simulink model "MGmono_rtiFPGASeparationFile"  (R2018b)
settings: Solver=FixedStepAuto  StartTime=0.0  StopTime=Inf  FixedStep=N*T  RelTol=1e-3
PostLoadFcn:
  | , if any(exist('dsrtsu_mdlpostloadfcn', 'file') ~= 0), dsrtsu_mdlpostloadfcn('Execute', bdroot); end,
InitFcn:
  | , if any(exist('dsmpb_private', 'file') ~= 0), dsmpb_private('dsmpb_mdlclblib', 'Init', bdroot); end,
values from neighbouring files (symbols this model uses):
  amp = 1    [param.m]
  fixedgain_i = 10*1000/(3*100)    (= 33.3333333333)    [param.m]
  fixedgain_vc1 = 10*10000/(3*100*2.5)    (= 133.333333333)    [param.m]
  fixedgain_vc2 = 10*10000/(3*100*2.5)    (= 133.333333333)    [param.m]
  fixedgain_vc3 = 10*22000/(3*100*2.5)    (= 293.333333333)    [param.m]
  fixedgain_vc4 = 10*22000/(3*100*2.5)    (= 293.333333333)    [param.m]
  fixedgain_vc5 = 10*22000/(3*100*2.5)    (= 293.333333333)    [param.m]
  freq = 50    [param.m]
  gain_iL1 = 1    [param.m]
  gain_iL2 = 1    [param.m]
  gain_iL3 = 1    [param.m]
  gain_iL4 = 1    [param.m]
  gain_vc1 = 1    [param.m]
  gain_vc2 = 1    [param.m]
  gain_vc3 = 1    [param.m]
  gain_vc4 = 1    [param.m]
  gain_vc5 = 1    [param.m]
  Ii = 10    [param.m]
  Ipv = 0.01    [param.m]
  Iv = 0.1    [param.m]
  Ki = 1e-7    (= 1e-07)    [param.m]
  Kp = 0.5    [param.m]
  maxd = N-1    (= 9)    [param.m]
  mind = 1    [param.m]
  N = 10    [param.m]
  offset_iL1 = 0.2    [param.m]
  offset_iL2 = 0.2    [param.m]
  offset_iL3 = -2e-3    (= -0.002)    [param.m]
  offset_iL4 = -2e-3    (= -0.002)    [param.m]
  offset_vc1 = -0.21    [param.m]
  offset_vc2 = -0.17    [param.m]
  offset_vc3 = 0.2    [param.m]
  offset_vc4 = -0.05    [param.m]
  offset_vc5 = -0.01    [param.m]
  Pi = 0.3    [param.m]
  Ppv = 0.05    [param.m]
  Pv = 0.01    [param.m]
  T = 6e-6    (= 6e-06)    [param.m]
  Tf = 1/1000    (= 0.001)    [param.m]
  Tfdc = 1/20    (= 0.05)    [param.m]
  v_dc_ref = 80    [param.m]
undefined symbols (not defined in the file or in its folder): DiscIntNeverNeededParam
libraries: xbsIndex_r4 x155, rti1202lib_adc_class1 x9, rtiproclib x7, simulink x6, rtifpgainterfacelib x1
(part 5 of 5)

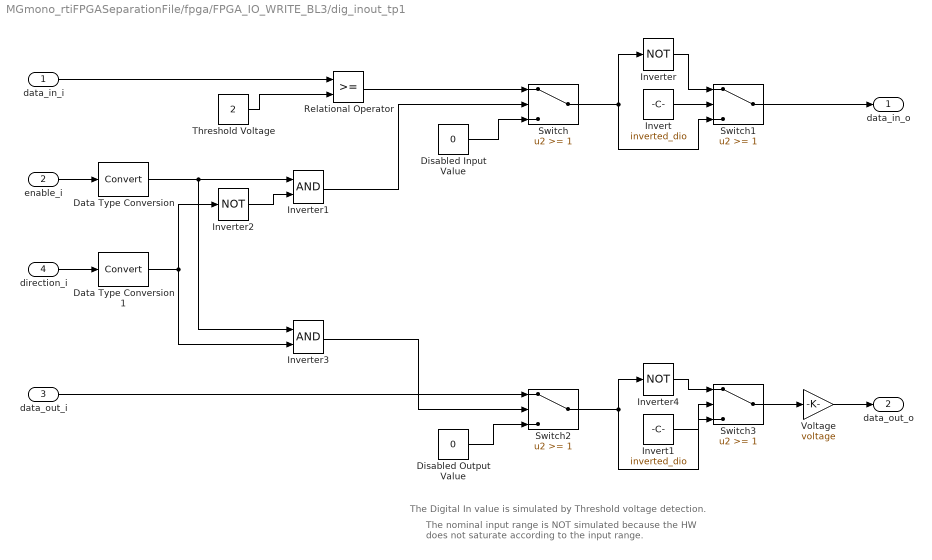
== system MGmono_rtiFPGASeparationFile/fpga/FPGA_IO_WRITE_BL3/dig_inout_tp1 ==
  note: The nominal input range is NOT simulated because
      | the HW does not saturate according to the input range.
  note: The Digital In value is simulated by Threshold voltage detection.
  data_in_i : Inport
  enable_i : Inport  Port=2
  data_out_i : Inport  Port=3
  direction_i : Inport  Port=4
  Data Type Conversion : DataTypeConversion
  Data Type Conversion1 : DataTypeConversion
  Disabled Input Value : Constant  Value=0
  Disabled Output Value : Constant  Value=0
  Invert : Constant  Value=inverted_dio
  Invert1 : Constant  Value=inverted_dio
  Inverter : Logic  Operator=NOT  AllPortsSameDT=off  OutDataTypeStr=boolean
  Inverter1 : Logic  AllPortsSameDT=off  OutDataTypeStr=boolean
  Inverter2 : Logic  Operator=NOT  AllPortsSameDT=off  OutDataTypeStr=boolean
  Inverter3 : Logic  AllPortsSameDT=off  OutDataTypeStr=boolean
  Inverter4 : Logic  Operator=NOT  AllPortsSameDT=off  OutDataTypeStr=boolean
  Relational Operator : RelationalOperator  OutDataTypeStr=boolean  RndMeth=Nearest
  Switch{,1..3} (4 alike) : Switch  Threshold=1
  Threshold Voltage : Constant  Value=2
  Voltage : Gain  Gain=voltage  ParamDataTypeStr=float('double')
  data_in_o : Outport
  data_out_o : Outport  Port=2
  wires:
  Voltage/1 -> data_out_o/1
  Data Type Conversion1/1 -> Inverter3/2, Inverter2/1
  Data Type Conversion/1 -> Inverter3/1, Inverter1/1
  Switch3/1 -> Voltage/1
  Switch2/1 -> Switch3/3, Inverter4/1
  Inverter4/1 -> Switch3/1
  Invert1/1 -> Switch3/2
  data_out_i/1 -> Switch2/1
  Inverter3/1 -> Switch2/2
  Disabled Output Value/1 -> Switch2/3
  Inverter2/1 -> Inverter1/2
  direction_i/1 -> Data Type Conversion1/1
  Inverter1/1 -> Switch/2
  enable_i/1 -> Data Type Conversion/1
  Switch/1 -> Switch1/3, Inverter/1
  Relational Operator/1 -> Switch/1
  Inverter/1 -> Switch1/1
  Invert/1 -> Switch1/2
  Switch1/1 -> data_in_o/1
  Disabled Input Value/1 -> Switch/3
  Threshold Voltage/1 -> Relational Operator/2
  data_in_i/1 -> Relational Operator/1

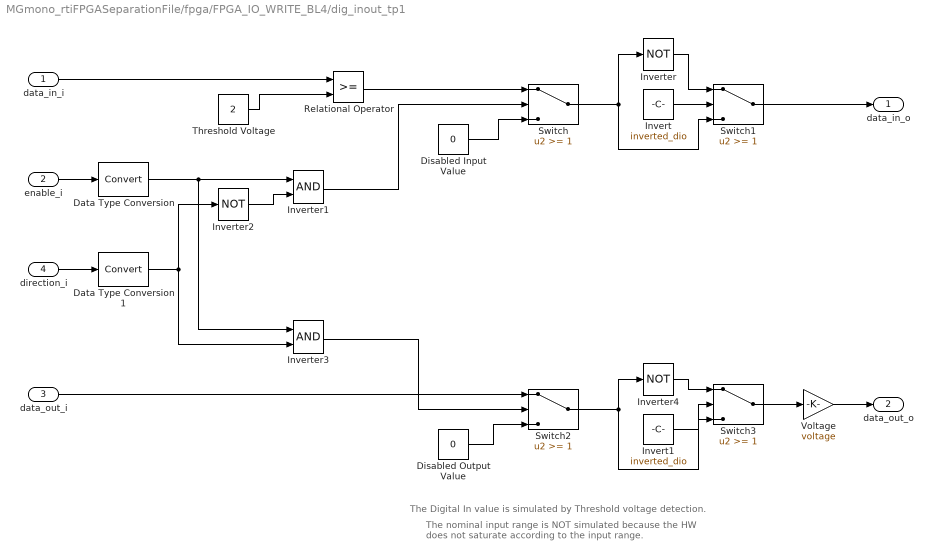
== system MGmono_rtiFPGASeparationFile/fpga/FPGA_IO_WRITE_BL4/dig_inout_tp1 ==
  note: The nominal input range is NOT simulated because
      | the HW does not saturate according to the input range.
  note: The Digital In value is simulated by Threshold voltage detection.
  data_in_i : Inport
  enable_i : Inport  Port=2
  data_out_i : Inport  Port=3
  direction_i : Inport  Port=4
  Data Type Conversion : DataTypeConversion
  Data Type Conversion1 : DataTypeConversion
  Disabled Input Value : Constant  Value=0
  Disabled Output Value : Constant  Value=0
  Invert : Constant  Value=inverted_dio
  Invert1 : Constant  Value=inverted_dio
  Inverter : Logic  Operator=NOT  AllPortsSameDT=off  OutDataTypeStr=boolean
  Inverter1 : Logic  AllPortsSameDT=off  OutDataTypeStr=boolean
  Inverter2 : Logic  Operator=NOT  AllPortsSameDT=off  OutDataTypeStr=boolean
  Inverter3 : Logic  AllPortsSameDT=off  OutDataTypeStr=boolean
  Inverter4 : Logic  Operator=NOT  AllPortsSameDT=off  OutDataTypeStr=boolean
  Relational Operator : RelationalOperator  OutDataTypeStr=boolean  RndMeth=Nearest
  Switch{,1..3} (4 alike) : Switch  Threshold=1
  Threshold Voltage : Constant  Value=2
  Voltage : Gain  Gain=voltage  ParamDataTypeStr=float('double')
  data_in_o : Outport
  data_out_o : Outport  Port=2
  wires:
  Voltage/1 -> data_out_o/1
  Data Type Conversion1/1 -> Inverter3/2, Inverter2/1
  Data Type Conversion/1 -> Inverter3/1, Inverter1/1
  Switch3/1 -> Voltage/1
  Switch2/1 -> Switch3/3, Inverter4/1
  Inverter4/1 -> Switch3/1
  Invert1/1 -> Switch3/2
  data_out_i/1 -> Switch2/1
  Inverter3/1 -> Switch2/2
  Disabled Output Value/1 -> Switch2/3
  Inverter2/1 -> Inverter1/2
  direction_i/1 -> Data Type Conversion1/1
  Inverter1/1 -> Switch/2
  enable_i/1 -> Data Type Conversion/1
  Switch/1 -> Switch1/3, Inverter/1
  Relational Operator/1 -> Switch/1
  Inverter/1 -> Switch1/1
  Invert/1 -> Switch1/2
  Switch1/1 -> data_in_o/1
  Disabled Input Value/1 -> Switch/3
  Threshold Voltage/1 -> Relational Operator/2
  data_in_i/1 -> Relational Operator/1

== system MGmono_rtiFPGASeparationFile/fpga/FPGA_IO_WRITE_BL5/dig_inout_tp1 ==
  note: The nominal input range is NOT simulated because
      | the HW does not saturate according to the input range.
  note: The Digital In value is simulated by Threshold voltage detection.
  data_in_i : Inport
  enable_i : Inport  Port=2
  data_out_i : Inport  Port=3
  direction_i : Inport  Port=4
  Data Type Conversion : DataTypeConversion
  Data Type Conversion1 : DataTypeConversion
  Disabled Input Value : Constant  Value=0
  Disabled Output Value : Constant  Value=0
  Invert : Constant  Value=inverted_dio
  Invert1 : Constant  Value=inverted_dio
  Inverter : Logic  Operator=NOT  AllPortsSameDT=off  OutDataTypeStr=boolean
  Inverter1 : Logic  AllPortsSameDT=off  OutDataTypeStr=boolean
  Inverter2 : Logic  Operator=NOT  AllPortsSameDT=off  OutDataTypeStr=boolean
  Inverter3 : Logic  AllPortsSameDT=off  OutDataTypeStr=boolean
  Inverter4 : Logic  Operator=NOT  AllPortsSameDT=off  OutDataTypeStr=boolean
  Relational Operator : RelationalOperator  OutDataTypeStr=boolean  RndMeth=Nearest
  Switch{,1..3} (4 alike) : Switch  Threshold=1
  Threshold Voltage : Constant  Value=2
  Voltage : Gain  Gain=voltage  ParamDataTypeStr=float('double')
  data_in_o : Outport
  data_out_o : Outport  Port=2
  wires:
  Voltage/1 -> data_out_o/1
  Data Type Conversion1/1 -> Inverter3/2, Inverter2/1
  Data Type Conversion/1 -> Inverter3/1, Inverter1/1
  Switch3/1 -> Voltage/1
  Switch2/1 -> Switch3/3, Inverter4/1
  Inverter4/1 -> Switch3/1
  Invert1/1 -> Switch3/2
  data_out_i/1 -> Switch2/1
  Inverter3/1 -> Switch2/2
  Disabled Output Value/1 -> Switch2/3
  Inverter2/1 -> Inverter1/2
  direction_i/1 -> Data Type Conversion1/1
  Inverter1/1 -> Switch/2
  enable_i/1 -> Data Type Conversion/1
  Switch/1 -> Switch1/3, Inverter/1
  Relational Operator/1 -> Switch/1
  Inverter/1 -> Switch1/1
  Invert/1 -> Switch1/2
  Switch1/1 -> data_in_o/1
  Disabled Input Value/1 -> Switch/3
  Threshold Voltage/1 -> Relational Operator/2
  data_in_i/1 -> Relational Operator/1

== system MGmono_rtiFPGASeparationFile/fpga/FPGA_XDATA_READ_BL1/phs_read_register ==
  note: Subsystem simulating the phs bus
      | access via RTLib functions.
  note: Subsystem simulating the communication
      | function specific behaviour. This is how the
      | FPGA framework driver takes effect on the data.
  data_i : Inport
  com_fct_model : Subsystem
  phs/rtlib_sim_model : Subsystem
  data_o : Outport
  data_new_o : Outport  Port=2
  wires:
  com_fct_model/2(data_new_o) -> data_new_o/1
  phs/rtlib_sim_model/1(data_o1) -> com_fct_model/1(data_i1)
  com_fct_model/1(data_o1) -> data_o/1
  data_i/1 -> phs/rtlib_sim_model/1(data_i1)

== system MGmono_rtiFPGASeparationFile/fpga/FPGA_XDATA_READ_BL2/phs_read_register ==
  note: Subsystem simulating the phs bus
      | access via RTLib functions.
  note: Subsystem simulating the communication
      | function specific behaviour. This is how the
      | FPGA framework driver takes effect on the data.
  data_i : Inport
  com_fct_model : Subsystem
  phs/rtlib_sim_model : Subsystem
  data_o : Outport
  data_new_o : Outport  Port=2
  wires:
  com_fct_model/2(data_new_o) -> data_new_o/1
  phs/rtlib_sim_model/1(data_o1) -> com_fct_model/1(data_i1)
  com_fct_model/1(data_o1) -> data_o/1
  data_i/1 -> phs/rtlib_sim_model/1(data_i1)

== system MGmono_rtiFPGASeparationFile/fpga/FPGA_XDATA_READ_BL3/phs_read_register ==
  note: Subsystem simulating the phs bus
      | access via RTLib functions.
  note: Subsystem simulating the communication
      | function specific behaviour. This is how the
      | FPGA framework driver takes effect on the data.
  data_i : Inport
  com_fct_model : Subsystem
  phs/rtlib_sim_model : Subsystem
  data_o : Outport
  data_new_o : Outport  Port=2
  wires:
  com_fct_model/2(data_new_o) -> data_new_o/1
  phs/rtlib_sim_model/1(data_o1) -> com_fct_model/1(data_i1)
  com_fct_model/1(data_o1) -> data_o/1
  data_i/1 -> phs/rtlib_sim_model/1(data_i1)

== system MGmono_rtiFPGASeparationFile/RTI Data/RTI Data Store/RTI Data Store/RTI Data Store ==
  RTI Data Store : Subsystem  mask(RTI_DATA_STORE){}
      mask help:
      | RTI Data Store Block. This block is used by RTI to store internal model dependent data. Deleting this block will result in data loss.
      |
      | NEVER DELETE, COPY, OR MODIFY THIS BLOCK!
      mask Help:
      | RTI Data Store Block. This block is used by RTI to store internal model dependent data. Deleting this block will result in data loss.
      | 
      | NEVER DELETE, COPY, OR MODIFY THIS BLOCK!
      mask Display: text(0.5, 0.5, ' ', 'HorizontalAlignment', 'center');

== system MGmono_rtiFPGASeparationFile/fpga/FPGA_INT_BL1/phs_interrupt/com_fct_model ==
  data_i1 : Inport
  data_o1 : Outport
  wires:
  data_i1/1 -> data_o1/1

== system MGmono_rtiFPGASeparationFile/fpga/FPGA_INT_BL1/phs_interrupt/phs//rtlib_sim_model ==
  note: - Detect the interrupt (rising edge).
      | - Generate function call.
  data_i1 : Inport
  Triggered Subsystem : Subsystem  TreatAsAtomicUnit=on
  data_o1 : Outport
  wires:
  Triggered Subsystem/1(Out1) -> data_o1/1
  data_i1/1 -> Triggered Subsystem/Trigger

== system MGmono_rtiFPGASeparationFile/fpga/FPGA_INT_BL2/phs_interrupt/com_fct_model ==
  data_i1 : Inport
  data_o1 : Outport
  wires:
  data_i1/1 -> data_o1/1

== system MGmono_rtiFPGASeparationFile/fpga/FPGA_INT_BL2/phs_interrupt/phs//rtlib_sim_model ==
  note: - Detect the interrupt (rising edge).
      | - Generate function call.
  data_i1 : Inport
  Triggered Subsystem : Subsystem  TreatAsAtomicUnit=on
  data_o1 : Outport
  wires:
  Triggered Subsystem/1(Out1) -> data_o1/1
  data_i1/1 -> Triggered Subsystem/Trigger

== system MGmono_rtiFPGASeparationFile/fpga/FPGA_INT_BL3/phs_interrupt/com_fct_model ==
  data_i1 : Inport
  data_o1 : Outport
  wires:
  data_i1/1 -> data_o1/1

== system MGmono_rtiFPGASeparationFile/fpga/FPGA_INT_BL3/phs_interrupt/phs//rtlib_sim_model ==
  note: - Detect the interrupt (rising edge).
      | - Generate function call.
  data_i1 : Inport
  Triggered Subsystem : Subsystem  TreatAsAtomicUnit=on
  data_o1 : Outport
  wires:
  Triggered Subsystem/1(Out1) -> data_o1/1
  data_i1/1 -> Triggered Subsystem/Trigger

== system MGmono_rtiFPGASeparationFile/fpga/FPGA_XDATA_READ_BL1/phs_read_register/com_fct_model ==
  note: - Register data is presented to the FPGA application without data adaptions.
      |
      | - Register group accesses are implicitly simulated by simulink: all FPGA
      | communication function interface blocks are simulated within one task
      | with a unique sample time --> in- and ouputs are sampled simultaneously
      | and therefore data consistency is guaranteed.
  data_i1 : Inport
  Data_New_Calc : Subsystem
  Zero-Order Hold : ZeroOrderHold  SampleTime=fpga_sample_time
  data_o1 : Outport
  data_new_o : Outport  Port=2
  wires:
  Zero-Order Hold/1 -> data_o1/1
  Data_New_Calc/1(Out1) -> data_new_o/1
  data_i1/1 -> Zero-Order Hold/1, Data_New_Calc/1(In1)

== system MGmono_rtiFPGASeparationFile/fpga/FPGA_XDATA_READ_BL1/phs_read_register/phs//rtlib_sim_model ==
  note: - The double to fixed-point conversion done by the XSG gateway behaves differently
      | than the conversion done by the RTLib C-code. Therefore the C-Code behaviour
      | is simulated via an s-function using the RTLib conversion technique including scaling and saturation.
  data_i1 : Inport
  S-Function : S-Function  FunctionName=DS1302_read_register  Parameters=mode;binaryPoint  SFunctionDeploymentMode=off  EnableBusSupport=off
  Zero-Order Hold : ZeroOrderHold  SampleTime=proc_sample_time
  data_o1 : Outport
  wires:
  Zero-Order Hold/1 -> S-Function/1
  S-Function/1 -> data_o1/1
  data_i1/1 -> Zero-Order Hold/1

== system MGmono_rtiFPGASeparationFile/fpga/FPGA_XDATA_READ_BL2/phs_read_register/com_fct_model ==
  note: - Register data is presented to the FPGA application without data adaptions.
      |
      | - Register group accesses are implicitly simulated by simulink: all FPGA
      | communication function interface blocks are simulated within one task
      | with a unique sample time --> in- and ouputs are sampled simultaneously
      | and therefore data consistency is guaranteed.
  data_i1 : Inport
  Data_New_Calc : Subsystem
  Zero-Order Hold : ZeroOrderHold  SampleTime=fpga_sample_time
  data_o1 : Outport
  data_new_o : Outport  Port=2
  wires:
  Zero-Order Hold/1 -> data_o1/1
  Data_New_Calc/1(Out1) -> data_new_o/1
  data_i1/1 -> Zero-Order Hold/1, Data_New_Calc/1(In1)

== system MGmono_rtiFPGASeparationFile/fpga/FPGA_XDATA_READ_BL2/phs_read_register/phs//rtlib_sim_model ==
  note: - The double to fixed-point conversion done by the XSG gateway behaves differently
      | than the conversion done by the RTLib C-code. Therefore the C-Code behaviour
      | is simulated via an s-function using the RTLib conversion technique including scaling and saturation.
  data_i1 : Inport
  S-Function : S-Function  FunctionName=DS1302_read_register  Parameters=mode;binaryPoint  SFunctionDeploymentMode=off  EnableBusSupport=off
  Zero-Order Hold : ZeroOrderHold  SampleTime=proc_sample_time
  data_o1 : Outport
  wires:
  Zero-Order Hold/1 -> S-Function/1
  S-Function/1 -> data_o1/1
  data_i1/1 -> Zero-Order Hold/1

== system MGmono_rtiFPGASeparationFile/fpga/FPGA_XDATA_READ_BL3/phs_read_register/com_fct_model ==
  note: - Register data is presented to the FPGA application without data adaptions.
      |
      | - Register group accesses are implicitly simulated by simulink: all FPGA
      | communication function interface blocks are simulated within one task
      | with a unique sample time --> in- and ouputs are sampled simultaneously
      | and therefore data consistency is guaranteed.
  data_i1 : Inport
  Data_New_Calc : Subsystem
  Zero-Order Hold : ZeroOrderHold  SampleTime=fpga_sample_time
  data_o1 : Outport
  data_new_o : Outport  Port=2
  wires:
  Zero-Order Hold/1 -> data_o1/1
  Data_New_Calc/1(Out1) -> data_new_o/1
  data_i1/1 -> Zero-Order Hold/1, Data_New_Calc/1(In1)

== system MGmono_rtiFPGASeparationFile/fpga/FPGA_XDATA_READ_BL3/phs_read_register/phs//rtlib_sim_model ==
  note: - The double to fixed-point conversion done by the XSG gateway behaves differently
      | than the conversion done by the RTLib C-code. Therefore the C-Code behaviour
      | is simulated via an s-function using the RTLib conversion technique including scaling and saturation.
  data_i1 : Inport
  S-Function : S-Function  FunctionName=DS1302_read_register  Parameters=mode;binaryPoint  SFunctionDeploymentMode=off  EnableBusSupport=off
  Zero-Order Hold : ZeroOrderHold  SampleTime=proc_sample_time
  data_o1 : Outport
  wires:
  Zero-Order Hold/1 -> S-Function/1
  S-Function/1 -> data_o1/1
  data_i1/1 -> Zero-Order Hold/1

== system MGmono_rtiFPGASeparationFile/RTI Data/RTI Data Store/RTI Data Store/RTI Data Store/RTI Data Store ==

== system MGmono_rtiFPGASeparationFile/fpga/FPGA_INT_BL1/phs_interrupt/phs//rtlib_sim_model/Triggered Subsystem ==
  Trigger : TriggerPort  VariantControl=(inherit)
  Function-Call Generator : simulink/Ports & Subsystems/Function-Call Generator  sample_time=-1  numberOfIterations=1
  Out1 : Outport
  wires:
  Function-Call Generator/1 -> Out1/1

== system MGmono_rtiFPGASeparationFile/fpga/FPGA_INT_BL2/phs_interrupt/phs//rtlib_sim_model/Triggered Subsystem ==
  Trigger : TriggerPort  VariantControl=(inherit)
  Function-Call Generator : simulink/Ports & Subsystems/Function-Call Generator  sample_time=-1  numberOfIterations=1
  Out1 : Outport
  wires:
  Function-Call Generator/1 -> Out1/1

== system MGmono_rtiFPGASeparationFile/fpga/FPGA_INT_BL3/phs_interrupt/phs//rtlib_sim_model/Triggered Subsystem ==
  Trigger : TriggerPort  VariantControl=(inherit)
  Function-Call Generator : simulink/Ports & Subsystems/Function-Call Generator  sample_time=-1  numberOfIterations=1
  Out1 : Outport
  wires:
  Function-Call Generator/1 -> Out1/1

== system MGmono_rtiFPGASeparationFile/fpga/FPGA_XDATA_READ_BL1/phs_read_register/com_fct_model/Data_New_Calc ==
  note: The new data flag is presented whenever the input data port is sampled.
      | The flag is set to 1 for one FPGA simulation step and reset to 0 for the
      | remaining FPGA simulation steps contained within one processor simulation step.
  In1 : Inport
  Add : Sum
  Constant : Constant  Value=fpga_sample_time  SampleTime=fpga_sample_time
  Constant1 : Constant  Value=0
  Divide : Product  Inputs=*/
  Divide1 : Product  Inputs=*/
  Math Function : Math  Operator=mod  SaturateOnIntegerOverflow=on
  Relational Operator : RelationalOperator  Operator===  OutDataTypeStr=boolean  RndMeth=Nearest
  Unit Delay1 : UnitDelay  InitialCondition=-1  SampleTime=-1
  Weighted Sample Time1 : SampleTimeMath  TsampMathOp=Ts Only
  Out1 : Outport
  wires:
  Constant/1 -> Divide1/2, Divide1/1, Divide/2
  Weighted Sample Time1/1 -> Divide/1
  Math Function/1 -> Relational Operator/1
  Relational Operator/1 -> Out1/1
  In1/1 -> Weighted Sample Time1/1
  Divide1/1 -> Add/1
  Unit Delay1/1 -> Add/2
  Add/1 -> Unit Delay1/1, Math Function/1
  Constant1/1 -> Relational Operator/2
  Divide/1 -> Math Function/2

== system MGmono_rtiFPGASeparationFile/fpga/FPGA_XDATA_READ_BL2/phs_read_register/com_fct_model/Data_New_Calc ==
  note: The new data flag is presented whenever the input data port is sampled.
      | The flag is set to 1 for one FPGA simulation step and reset to 0 for the
      | remaining FPGA simulation steps contained within one processor simulation step.
  In1 : Inport
  Add : Sum
  Constant : Constant  Value=fpga_sample_time  SampleTime=fpga_sample_time
  Constant1 : Constant  Value=0
  Divide : Product  Inputs=*/
  Divide1 : Product  Inputs=*/
  Math Function : Math  Operator=mod  SaturateOnIntegerOverflow=on
  Relational Operator : RelationalOperator  Operator===  OutDataTypeStr=boolean  RndMeth=Nearest
  Unit Delay1 : UnitDelay  InitialCondition=-1  SampleTime=-1
  Weighted Sample Time1 : SampleTimeMath  TsampMathOp=Ts Only
  Out1 : Outport
  wires:
  Constant/1 -> Divide1/2, Divide1/1, Divide/2
  Weighted Sample Time1/1 -> Divide/1
  Math Function/1 -> Relational Operator/1
  Relational Operator/1 -> Out1/1
  In1/1 -> Weighted Sample Time1/1
  Divide1/1 -> Add/1
  Unit Delay1/1 -> Add/2
  Add/1 -> Unit Delay1/1, Math Function/1
  Constant1/1 -> Relational Operator/2
  Divide/1 -> Math Function/2

== system MGmono_rtiFPGASeparationFile/fpga/FPGA_XDATA_READ_BL3/phs_read_register/com_fct_model/Data_New_Calc ==
  note: The new data flag is presented whenever the input data port is sampled.
      | The flag is set to 1 for one FPGA simulation step and reset to 0 for the
      | remaining FPGA simulation steps contained within one processor simulation step.
  In1 : Inport
  Add : Sum
  Constant : Constant  Value=fpga_sample_time  SampleTime=fpga_sample_time
  Constant1 : Constant  Value=0
  Divide : Product  Inputs=*/
  Divide1 : Product  Inputs=*/
  Math Function : Math  Operator=mod  SaturateOnIntegerOverflow=on
  Relational Operator : RelationalOperator  Operator===  OutDataTypeStr=boolean  RndMeth=Nearest
  Unit Delay1 : UnitDelay  InitialCondition=-1  SampleTime=-1
  Weighted Sample Time1 : SampleTimeMath  TsampMathOp=Ts Only
  Out1 : Outport
  wires:
  Constant/1 -> Divide1/2, Divide1/1, Divide/2
  Weighted Sample Time1/1 -> Divide/1
  Math Function/1 -> Relational Operator/1
  Relational Operator/1 -> Out1/1
  In1/1 -> Weighted Sample Time1/1
  Divide1/1 -> Add/1
  Unit Delay1/1 -> Add/2
  Add/1 -> Unit Delay1/1, Math Function/1
  Constant1/1 -> Relational Operator/2
  Divide/1 -> Math Function/2

== matlab function MGmono_rtiFPGASeparationFile/MPPT_system/MATLAB Function ==
  data: v_pv input; v_PandO output; i input; v_dc input; P output
function [v_PandO, P] = MPPT(v_pv,i, v_dc)
persistent P_ant v_ref v_ant contador vdc_ant

if isempty(P_ant)
    contador = 0;
    P_ant = 24;
    v_ref = 12;
    v_ant = 12;
    vdc_ant = 80;
end


P = v_pv*i;
contador = contador + 1;
if contador == 100
    contador = 1;
end

if contador == 1
    delta = P-P_ant;
    if (abs(delta) < 0.1)
    elseif delta > 0
            if v_pv>v_ant
                v_ref = v_ref+.1;
            else
                v_ref = v_ref-.1;
            end
    else
            if v_pv>v_ant
                v_ref = v_ref-.1;
            else
                v_ref = v_ref+.1;
            end
    end
    if v_ref>19
        v_ref = 19;
    end
    if v_ref<5
        v_ref = 5;
    end
    P_ant = P;
    v_ant = v_pv;
    vdc_ant = v_dc;
end

v_PandO = v_ref;
